simulink model "SPYNX_Simulink_17a"  (R2017a)
settings: Solver=VariableStepAuto  StartTime=0.0  StopTime=2  MaxStep=.00001  RelTol=1e-3  EnableMultiTasking=on
libraries: simulink x6
settings Model: PauseTimes=0.053  Creator=ga53xem  LastModifiedBy=ga53xem
settings DataIOCC: InspectSignalLogs=on
settings OptimizationCC: LifeSpan=inf
settings DebuggingCC: SFUnexpectedBacktrackingDiag=warning  SFNoUnconditionalDefaultTransitionDiag=warning  SFExecutionAtInitializationDiag=none
settings SFSimCC: SimCustomHeaderCode="#include \"FCSMPC_2.0.h\""  SimUserSources=FCSMPC_2.0.c
settings GRTTargetCC: TargetLangStandard=C89/C90 (ANSI)  GeneratePreprocessorConditionals=Disable all
settings ConfigComp: CovMetricSettings=dw  CovHtmlReporting=on  CovSaveCumulativeToWorkspaceVar=on  CovSaveSingleToWorkspaceVar=on  CovExternalEMLEnable=off

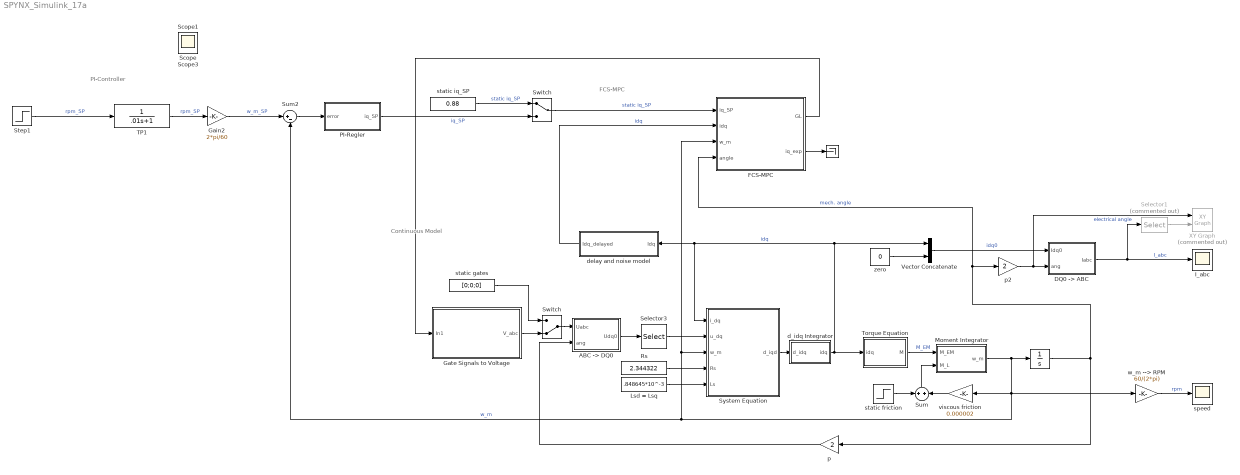
== system SPYNX_Simulink_17a ==
  note: PI-Controller
  note: FCS-MPC
  note: Continuous Model
  "  " : Terminator
  "   " : Integrator  WrapState=on  WrappedStateUpperValue=2*pi  WrappedStateLowerValue=0  ContinuousStateAttributes='angle_m'
  " Switch" : ManualSwitch
  "ABC -> DQ0" : MATLAB Function  TreatAsAtomicUnit=on
  "DQ0 -> ABC" : MATLAB Function  TreatAsAtomicUnit=on
  FCS-MPC : Subsystem  TreatAsAtomicUnit=on  SystemSampleTime=5.85e-6
  Gain2 : Gain  Gain=2*pi/60
  Gate Signals to Voltage : Subsystem
  I_abc : Scope
  Lsd = Lsq : Constant  Value=.848645*10^-3  OutDataTypeStr=double
  Moment Integrator : Subsystem
  PI-Regler : Subsystem
  Rs : Constant  Value=2.344322  OutDataTypeStr=double
  Selector1 : Selector  Commented=on  InputPortWidth=3  IndexOptions=Index vector (dialog)  Indices=[2]  OutputSizes=1
  Selector3 : Selector  InputPortWidth=3  IndexOptions=Index vector (dialog)  Indices=[1,2]  OutputSizes=1
  Step1 : Step  Before=4000  After=5000  SampleTime=0
  Sum : Sum  Inputs=+|+
  Sum2 : Sum  Inputs=|+-
  Switch : ManualSwitch  CurrentSetting=0
  System Equation : MATLAB Function  TreatAsAtomicUnit=on
  TP1 : TransferFcn  Denominator=[.01 1]
  Torque Equation : Subsystem
  Vector Concatenate : Concatenate
  XY Graph : simulink/Sinks/XY Graph  Commented=on  xmin=0  xmax=4*pi  ymin=-1  ymax=1  st=-1
  d_idq Integrator : Subsystem
  delay and noise model : Subsystem  TreatAsAtomicUnit=on
  p : Gain  Gain=2
  p2 : Gain  Gain=2
  speed : Scope
  static friction : Step  Time=0  After=.00058  SampleTime=0
  static gates : Constant  Value=[0;0;0]  OutDataTypeStr=double
  static iq_SP : Constant  Value=0.88  OutDataTypeStr=double
  viscous friction : Gain  Gain=0.000002
  w_m --> RPM : Gain  Gain=60/(2*pi)
  zero : Constant  Value=0  OutDataTypeStr=double
  Scope : Scope
  Scope1 : Scope
  Scope3 : Scope
  wires:
  "DQ0 -> ABC"/1(Iabc) -> I_abc/1, Selector1/1  "I_abc"
  zero/1 -> Vector Concatenate/2
  Vector Concatenate/1 -> "DQ0 -> ABC"/1(Idq0)  "idq0"
  p2/1 -> XY Graph/1, "DQ0 -> ABC"/2(ang)  "electrical angle"
  Sum/1 -> Moment Integrator/2(M_L)
  viscous friction/1 -> Sum/2
  Torque Equation/1(M) -> Moment Integrator/1(M_EM)  "M_EM"
  Lsd = Lsq/1 -> System Equation/5(Ls)
  static friction/1 -> Sum/1
  Selector3/1 -> System Equation/2(u_dq)
  Moment Integrator/1(w_m) -> "   "/1, w_m --> RPM/1, Sum2/2, FCS-MPC/3(w_m), System Equation/3(w_m), viscous friction/1  "w_m"
  System Equation/1(d_iqd) -> d_idq Integrator/1(d_idq)
  "ABC -> DQ0"/1(Udq0) -> Selector3/1
  w_m --> RPM/1 -> speed/1  "rpm"
  Rs/1 -> System Equation/4(Rs)
  p/1 -> "ABC -> DQ0"/2(ang)
  "   "/1 -> FCS-MPC/4(angle), p2/1, p/1  "mech. angle"
  Selector1/1 -> XY Graph/2
  d_idq Integrator/1(idq) -> Vector Concatenate/1, System Equation/1(i_dq), delay and noise model/1(Idq), Torque Equation/1(idq)  "idq"
  Gate Signals to Voltage/1(V_abc) -> Switch/2
  static gates/1 -> Switch/1
  FCS-MPC/1(GL) -> Gate Signals to Voltage/1(In1)
  delay and noise model/1(Idq_delayed) -> FCS-MPC/2(idq)  "idq"
  FCS-MPC/2(iq_exp) -> "  "/1
  " Switch"/1 -> FCS-MPC/1(iq_SP)  "static iq_SP"
  Sum2/1 -> PI-Regler/1(error)
  TP1/1 -> Gain2/1  "rpm_SP"
  Gain2/1 -> Sum2/1  "w_m_SP"
  PI-Regler/1(iq_SP) -> " Switch"/2  "iq_SP"
  Step1/1 -> TP1/1  "rpm_SP"
  static iq_SP/1 -> " Switch"/1  "static iq_SP"
  Switch/1 -> "ABC -> DQ0"/1(Uabc)

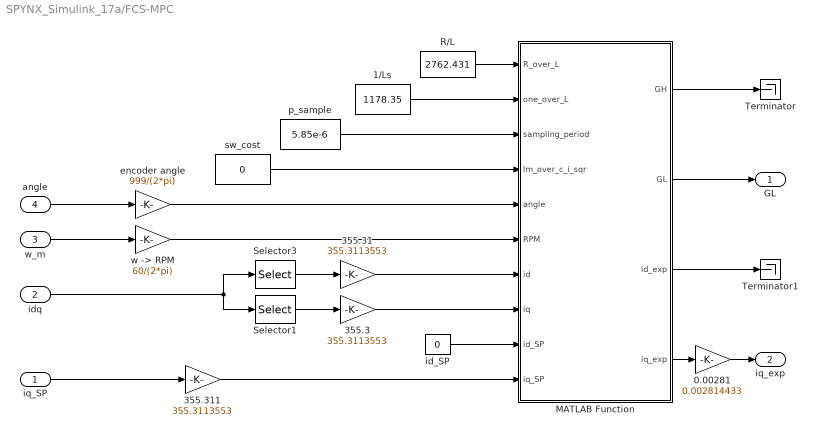
== system SPYNX_Simulink_17a/FCS-MPC ==
  iq_SP : Inport
  idq : Inport  Port=2
  w_m : Inport  Port=3
  angle : Inport  Port=4
  "0.00281 " : Gain  Gain=0.002814433
  "1/Ls\t" : Constant  Value=1178.35  OutDataTypeStr=single
  "355.3 " : Gain  Gain=355.3113553
  355.31 : Gain  Gain=355.3113553
  355.311 : Gain  Gain=355.3113553
  MATLAB Function : MATLAB Function  TreatAsAtomicUnit=on
  R/L : Constant  Value=2762.431  OutDataTypeStr=single
  Selector1 : Selector  InputPortWidth=2  IndexOptions=Index vector (dialog)  Indices=[2]  OutputSizes=1
  Selector3 : Selector  InputPortWidth=2  IndexOptions=Index vector (dialog)  Indices=[1]  OutputSizes=1
  Terminator : Terminator
  Terminator1 : Terminator
  encoder angle : Gain  Gain=999/(2*pi)
  id_SP : Constant  Value=0  OutDataTypeStr=int16
  p_sample : Constant  Value=5.85e-6  OutDataTypeStr=single
  sw_cost : Constant  Value=0  OutDataTypeStr=uint16
  "w -> RPM" : Gain  Gain=60/(2*pi)
  GL : Outport
  iq_exp : Outport  Port=2
  wires:
  R/L/1 -> MATLAB Function/1(R_over_L)
  p_sample/1 -> MATLAB Function/3(sampling_period)
  "1/Ls\t"/1 -> MATLAB Function/2(one_over_L)
  id_SP/1 -> MATLAB Function/9(id_SP)
  iq_SP/1 -> 355.311/1
  Selector1/1 -> "355.3 "/1
  Selector3/1 -> 355.31/1
  w_m/1 -> "w -> RPM"/1
  MATLAB Function/2(GL) -> GL/1
  "w -> RPM"/1 -> MATLAB Function/6(RPM)
  355.311/1 -> MATLAB Function/10(iq_SP)
  angle/1 -> encoder angle/1
  encoder angle/1 -> MATLAB Function/5(angle)
  idq/1 -> Selector1/1, Selector3/1
  MATLAB Function/1(GH) -> Terminator/1
  MATLAB Function/4(iq_exp) -> "0.00281 "/1
  MATLAB Function/3(id_exp) -> Terminator1/1
  "0.00281 "/1 -> iq_exp/1
  355.31/1 -> MATLAB Function/7(id)
  "355.3 "/1 -> MATLAB Function/8(iq)
  sw_cost/1 -> MATLAB Function/4(lm_over_c_i_sqr)

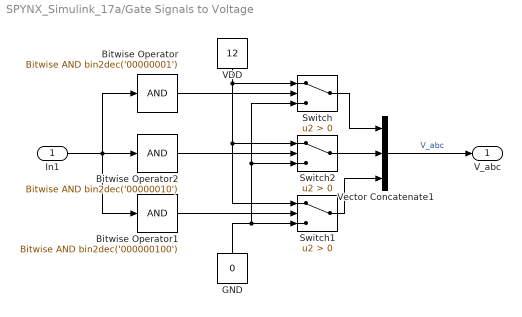
== system SPYNX_Simulink_17a/Gate Signals to Voltage ==
  In1 : Inport
  Bitwise Operator : simulink/Logic and Bit Operations/Bitwise Operator  logicop=AND  UseBitMask=on  BitMask=bin2dec('00000001')  BitMaskRealWorld=Stored Integer
  Bitwise Operator1 : simulink/Logic and Bit Operations/Bitwise Operator  logicop=AND  UseBitMask=on  BitMask=bin2dec('000000100')  BitMaskRealWorld=Stored Integer
  Bitwise Operator2 : simulink/Logic and Bit Operations/Bitwise Operator  logicop=AND  UseBitMask=on  BitMask=bin2dec('00000010')  BitMaskRealWorld=Stored Integer
  GND : Constant  Value=0  OutDataTypeStr=double
  Switch : Switch  Criteria=u2 > Threshold
  Switch1 : Switch  Criteria=u2 > Threshold
  Switch2 : Switch  Criteria=u2 > Threshold
  VDD : Constant  Value=12  OutDataTypeStr=double
  Vector Concatenate1 : Concatenate  NumInputs=3
  V_abc : Outport
  wires:
  Switch/1 -> Vector Concatenate1/1
  GND/1 -> Switch/3, Switch2/3, Switch1/3
  Bitwise Operator/1 -> Switch/2
  VDD/1 -> Switch2/1, Switch1/1, Switch/1
  Bitwise Operator1/1 -> Switch1/2
  Switch2/1 -> Vector Concatenate1/2
  Switch1/1 -> Vector Concatenate1/3
  Bitwise Operator2/1 -> Switch2/2
  Vector Concatenate1/1 -> V_abc/1  "V_abc"
  In1/1 -> Bitwise Operator1/1, Bitwise Operator2/1, Bitwise Operator/1

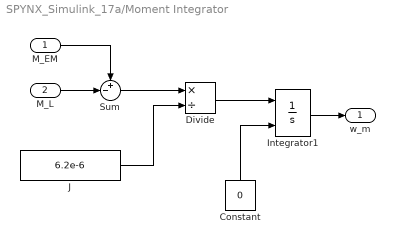
== system SPYNX_Simulink_17a/Moment Integrator ==
  M_EM : Inport
  M_L : Inport  Port=2
  Constant : Constant  Value=0
  Divide : Product  Inputs=*/
  Integrator1 : Integrator  InitialConditionSource=external
  J : Constant  Value=6.2e-6  OutDataTypeStr=double
  Sum : Sum  Inputs=+-|
  w_m : Outport
  wires:
  J/1 -> Divide/2
  Divide/1 -> Integrator1/1
  M_EM/1 -> Sum/1
  Integrator1/1 -> w_m/1
  M_L/1 -> Sum/2
  Sum/1 -> Divide/1
  Constant/1 -> Integrator1/2

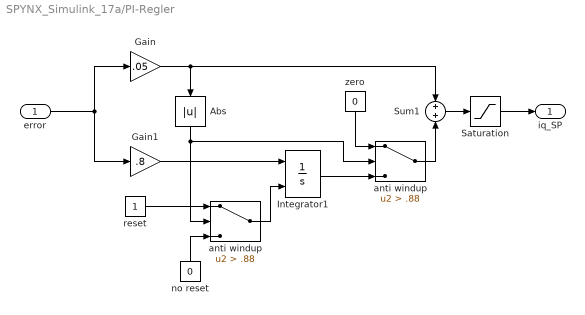
== system SPYNX_Simulink_17a/PI-Regler ==
  error : Inport
  Abs : Abs
  Gain : Gain  Gain=.05
  Gain1 : Gain  Gain=.8
  Integrator1 : Integrator  ExternalReset=falling  LimitOutput=on  UpperSaturationLimit=.88  LowerSaturationLimit=-.88
  Saturation : Saturate  UpperLimit=0.88  LowerLimit=-0.88
  Sum1 : Sum  Inputs=+|+
  anti windup : Switch  Criteria=u2 > Threshold  Threshold=.88
  "anti windup " : Switch  Criteria=u2 > Threshold  Threshold=.88
  no reset : Constant  Value=0  OutDataTypeStr=double
  reset : Constant  OutDataTypeStr=double
  zero : Constant  Value=0  OutDataTypeStr=double
  iq_SP : Outport
  wires:
  Saturation/1 -> iq_SP/1
  error/1 -> Gain/1, Gain1/1
  no reset/1 -> anti windup/3
  "anti windup "/1 -> Sum1/2
  Gain1/1 -> Integrator1/1
  reset/1 -> anti windup/1
  Sum1/1 -> Saturation/1
  anti windup/1 -> Integrator1/2
  Gain/1 -> Abs/1, Sum1/1
  Abs/1 -> anti windup/2, "anti windup "/2
  Integrator1/1 -> "anti windup "/3
  zero/1 -> "anti windup "/1

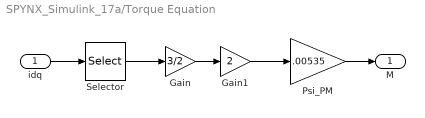
== system SPYNX_Simulink_17a/Torque Equation ==
  idq : Inport
  Gain : Gain  Gain=3/2
  Gain1 : Gain  Gain=2
  Psi_PM : Gain  Gain=.00535
  Selector : Selector  InputPortWidth=2  IndexOptions=Starting index (dialog)  Indices=[2]  OutputSizes=1
  M : Outport
  wires:
  Gain/1 -> Gain1/1
  Selector/1 -> Gain/1
  Gain1/1 -> Psi_PM/1
  Psi_PM/1 -> M/1
  idq/1 -> Selector/1

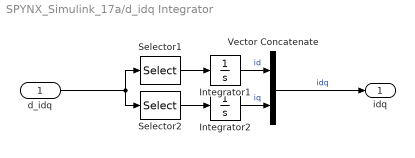
== system SPYNX_Simulink_17a/d_idq Integrator ==
  d_idq : Inport
  Integrator1 : Integrator
  Integrator2 : Integrator
  Selector1 : Selector  InputPortWidth=2  IndexOptions=Starting index (dialog)  Indices=[1]  OutputSizes=1
  Selector2 : Selector  InputPortWidth=2  IndexOptions=Starting index (dialog)  Indices=[2]  OutputSizes=1
  Vector Concatenate : Concatenate
  idq : Outport
  wires:
  Integrator1/1 -> Vector Concatenate/1  "id"
  Selector2/1 -> Integrator2/1
  Vector Concatenate/1 -> idq/1  "idq"
  Integrator2/1 -> Vector Concatenate/2  "iq"
  Selector1/1 -> Integrator1/1
  d_idq/1 -> Selector1/1, Selector2/1

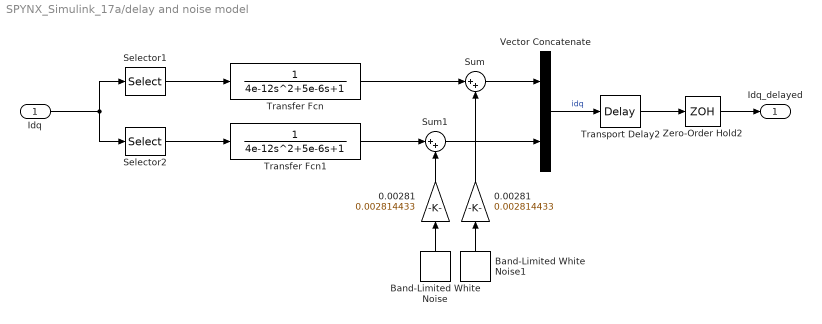
== system SPYNX_Simulink_17a/delay and noise model ==
  Idq : Inport
  0.00281 : Gain  Gain=0.002814433
  "0.00281 " : Gain  Gain=0.002814433
  Band-Limited White Noise : simulink/Sources/Band-Limited White Noise  Cov=[.0001]  Ts=6.4e-6  seed=[23341]
  Band-Limited White Noise1 : simulink/Sources/Band-Limited White Noise  Cov=[.0001]  Ts=6.4e-6  seed=[23341]
  Selector1 : Selector  InputPortWidth=2  IndexOptions=Starting index (dialog)  Indices=[1]  OutputSizes=1
  Selector2 : Selector  InputPortWidth=2  IndexOptions=Starting index (dialog)  Indices=[2]  OutputSizes=1
  Sum : Sum  Inputs=|++
  Sum1 : Sum  Inputs=|++
  Transfer Fcn : TransferFcn  Denominator=[4e-12 5e-6 1]
  Transfer Fcn1 : TransferFcn  Denominator=[4e-12 5e-6 1]
  Transport Delay2 : TransportDelay  DelayTime=1e-6
  Vector Concatenate : Concatenate
  Zero-Order Hold2 : ZeroOrderHold  SampleTime=1.6e-6
  Idq_delayed : Outport
  wires:
  Selector1/1 -> Transfer Fcn/1
  Selector2/1 -> Transfer Fcn1/1
  Vector Concatenate/1 -> Transport Delay2/1  "idq"
  Idq/1 -> Selector2/1, Selector1/1
  Transfer Fcn1/1 -> Sum1/1
  Transfer Fcn/1 -> Sum/1
  Sum/1 -> Vector Concatenate/1
  Sum1/1 -> Vector Concatenate/2
  Band-Limited White Noise/1 -> "0.00281 "/1
  Band-Limited White Noise1/1 -> 0.00281/1
  0.00281/1 -> Sum/2
  "0.00281 "/1 -> Sum1/2
  Zero-Order Hold2/1 -> Idq_delayed/1
  Transport Delay2/1 -> Zero-Order Hold2/1

== matlab function SPYNX_Simulink_17a/FCS-MPC/MATLAB Function ==
  data: R_over_L input; GH output; one_over_L input; sampling_period input; lm_over_c_i_sqr input; angle input; RPM input; id input; iq input; id_SP input; iq_SP input; GL output; id_exp output; iq_exp output
function [GH, GL, id_exp, iq_exp] = fcn(R_over_L, one_over_L, sampling_period, lm_over_c_i_sqr, angle, RPM, id, iq, id_SP, iq_SP)
GH = uint8(0);
GL = uint8(0);
id_exp = int16(0);
iq_exp = int16(0);
persistent RPM_m;   % persistant vatriables are needed to model the execution...
persistent id_m;    % ... delay of the code. Without this the execution time...
persistent iq_m;    % ... is zero.
if isempty(RPM_m)
    RPM_m = 0;
    id_m = 0;
    iq_m = 0;
end
coder.ceval('FCSMPC', R_over_L, one_over_L, sampling_period, uint16(lm_over_c_i_sqr),...
                    int16(angle), int16(RPM_m), int16(id_m), int16(iq_m), int16(id_SP), int16(iq_SP), ...
                    coder.wref(GH), coder.wref(GL), coder.wref(id_exp), coder.wref(iq_exp));
RPM_m = RPM;
id_m = id;
iq_m = iq;

== matlab function SPYNX_Simulink_17a/System Equation ==
  data: i_dq input; d_iqd output; u_dq input; w_m input; Rs input; Ls input
function d_iqd = fcn(i_dq, u_dq, w_m, Rs, Ls)

d_iqd = [[-Rs/Ls, w_m*2]; 
        [-w_m*2, -Rs/Ls]]*i_dq + [[1/Ls, 0];
                                  [0, 1/Ls]]*u_dq - [   0   ;
                                                     w_m*10.3472]; % RPM*385 = w_m/2pi*60*385*ci = w_m*10.3472
end

== matlab function SPYNX_Simulink_17a/ABC -> DQ0 ==
  data: Uabc input; Udq0 output; ang input
function Udq0 = fcn(Uabc, ang)
Udq0 = 2/3* [ cos(ang),  cos(ang-2*pi/3),  cos(ang-4*pi/3); 
             -sin(ang), -sin(ang-2*pi/3), -sin(ang-4*pi/3);
               .5,             .5,                 .5     ] * Uabc;

== matlab function SPYNX_Simulink_17a/DQ0 -> ABC ==
  data: Idq0 input; Iabc output; ang input
function Iabc = fcn(Idq0, ang)
Iabc = [cos(ang),       -sin(ang),        1;
        cos(ang-2*pi/3),-sin(ang-2*pi/3), 1;
        cos(ang-4*pi/3),-sin(ang-4*pi/3), 1] * Idq0;
